simulink model "ship_template"  (R2021b)
settings: Solver=ode23t  StartTime=0.0  StopTime=60*2  MaxStep=0.1  RelTol=1e-3  AbsTol=1e-3
model workspace (MAT data in the model file):
  L = 1.2
  W = 1.2
undefined symbols (not defined in the file or in its folder): blue, blue0, blue1, blue2, centre, green, green0, green1, green2, left, Left, llx, lly, Mid, red, red0, red1, red2, right, Right, ulx, uly, X, Y, Z
libraries: sm_lib x278, nesl_utility x68, fl_lib x58, simulink x12, ee_lib x3, sdl_lib x3
(part 3 of 8)

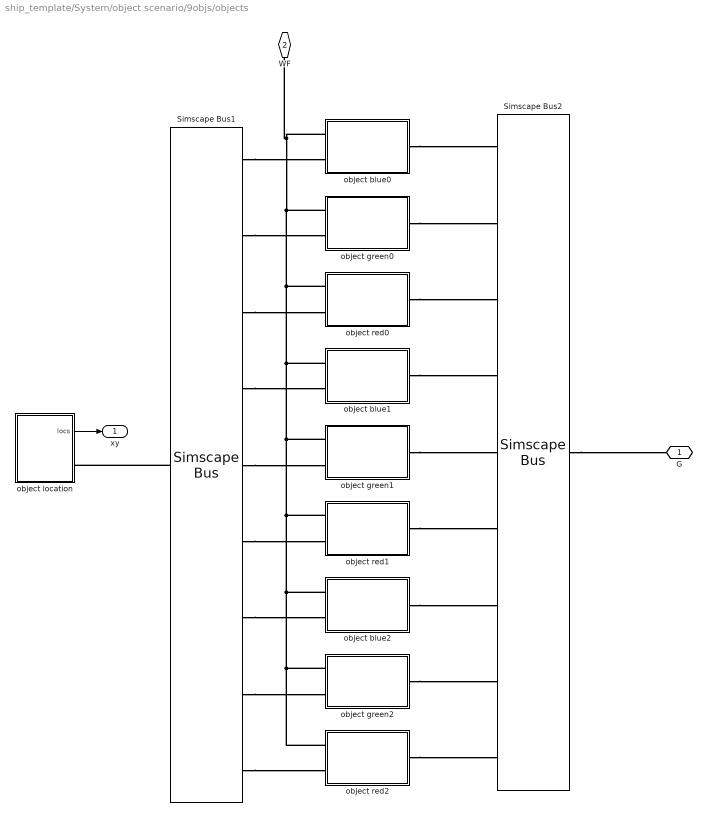
== system ship_template/System/object scenario/9objs/objects ==
  Simscape Bus1 : SimscapeBus  HierarchyStrings=blue0;green0;red0;blue1;green1;red1;blue2;green2;red2
  Simscape Bus2 : SimscapeBus  HierarchyStrings=blue0;green0;red0;blue1;green1;red1;blue2;green2;red2
  object blue0 : Subsystem  mask{x0=object_locs(1,1), y0=object_locs(1,2), color=[0.1 0.1 0.8]}
      mask prompts: x0 "Initial position x (m)"; y0 "Initial position y (m)"; color "Colour (RGB)"
  object blue1 : Subsystem  mask{x0=object_locs(4,1), y0=object_locs(4,2), color=[0.1 0.1 0.8]}
      mask prompts: x0 "Initial position x (m)"; y0 "Initial position y (m)"; color "Colour (RGB)"
  object blue2 : Subsystem  mask{x0=object_locs(7,1), y0=object_locs(7,2), color=[0.1 0.1 0.8]}
      mask prompts: x0 "Initial position x (m)"; y0 "Initial position y (m)"; color "Colour (RGB)"
  object green0 : Subsystem  mask{x0=object_locs(2,1), y0=object_locs(2,2), color=[0.1 0.8 0.1]}
      mask prompts: x0 "Initial position x (m)"; y0 "Initial position y (m)"; color "Colour (RGB)"
  object green1 : Subsystem  mask{x0=object_locs(5,1), y0=object_locs(5,2), color=[0.1 0.8 0.1]}
      mask prompts: x0 "Initial position x (m)"; y0 "Initial position y (m)"; color "Colour (RGB)"
  object green2 : Subsystem  mask{x0=object_locs(8,1), y0=object_locs(8,2), color=[0.1 0.8 0.1]}
      mask prompts: x0 "Initial position x (m)"; y0 "Initial position y (m)"; color "Colour (RGB)"
  object location : Subsystem  mask{Xhome=0, Yhome=0, homeRadius=0.1}
      mask prompts: Xhome "X home (m)"; Yhome "Y home (m)"; homeRadius "Home radius (m)"
  object red0 : Subsystem  mask{x0=object_locs(3,1), y0=object_locs(3,2), color=[0.8 0.1 0.1]}
      mask prompts: x0 "Initial position x (m)"; y0 "Initial position y (m)"; color "Colour (RGB)"
  object red1 : Subsystem  mask{x0=object_locs(6,1), y0=object_locs(6,2), color=[0.8 0.1 0.1]}
      mask prompts: x0 "Initial position x (m)"; y0 "Initial position y (m)"; color "Colour (RGB)"
  object red2 : Subsystem  mask{x0=object_locs(9,1), y0=object_locs(9,2), color=[0.8 0.1 0.1]}
      mask prompts: x0 "Initial position x (m)"; y0 "Initial position y (m)"; color "Colour (RGB)"
  G : PMIOPort  Side=Right
  WF : PMIOPort  Port=2  Side=Left
  xy : Outport
  wires:
  object location/1(locs) -> xy/1
  connections:
  object red0/RConn1 -- Simscape Bus2/LConn3
  object blue0/LConn1 -- object red2/LConn1 -- object green2/LConn1 -- object blue2/LConn1 -- object red1/LConn1 -- object green1/LConn1 -- object blue1/LConn1 -- object red0/LConn1 -- object green0/LConn1 -- WF/RConn1
  object blue0/RConn1 -- Simscape Bus2/LConn1
  object green0/RConn1 -- Simscape Bus2/LConn2
  Simscape Bus2/RConn1 -- G/RConn1
  Simscape Bus1/RConn1 -- object location/RConn1
  object blue1/RConn1 -- Simscape Bus2/LConn4
  object green1/RConn1 -- Simscape Bus2/LConn5
  object red1/RConn1 -- Simscape Bus2/LConn6
  object blue2/RConn1 -- Simscape Bus2/LConn7
  object green2/RConn1 -- Simscape Bus2/LConn8
  object red2/RConn1 -- Simscape Bus2/LConn9
  Simscape Bus1/LConn1 -- object blue0/LConn2
  Simscape Bus1/LConn2 -- object green0/LConn2
  Simscape Bus1/LConn3 -- object red0/LConn2
  Simscape Bus1/LConn4 -- object blue1/LConn2
  Simscape Bus1/LConn5 -- object green1/LConn2
  Simscape Bus1/LConn6 -- object red1/LConn2
  Simscape Bus1/LConn7 -- object blue2/LConn2
  Simscape Bus1/LConn8 -- object green2/LConn2
  Simscape Bus1/LConn9 -- object red2/LConn2

== system ship_template/System/propulsion and steering/one propeller and rudder (experimental)/Servo Rudder Mechanism ==
  angle : Inport
  Drag : Subsystem  mask{Cd=CdRud, L=LengthRudmm, D=DepthRudmm, rho=densityWorkingFluid}
      mask prompts: Cd "Drag coefficient"; L "Submerged Rudder Length (mm)"; D "Submerged Rudder Depth (mm)"; rho "Density"
  Pin : sm_lib/Body Elements/Cylindrical Solid  GraphicAmbientColor=[0.15 0.15 0.15 1.0]  BasedOnType=Density  CenterOfMass=[0 0 0]  CenterOfMassUnits=m  GraphicDiffuseColor=[1.0 1.0 1.0]  CylinderLength=5  CylinderLengthUnits=mm  CylinderRadius=3  CylinderRadiusUnits=mm  Density=1000  DensityUnits=kg/m^3  DoExposeReferenceFrame=on  GraphicEmissiveColor=[0.0 0.0 0.0 1.0]  ExportEntireGeometry=off  SerializedFrames=<Frames/>  MarkerShape=Sphere  MarkerSize=10  GraphicType=FromGeometry  InertiaType=CalculateFromGeometry  Mass=1  MassUnits=kg  MomentsOfInertia=[1 1 1]  MomentsOfInertiaUnits=kg*m^2  GraphicOpacity=1.0  ProductsOfInertia=[0 0 0]  ProductsOfInertiaUnits=kg*m^2  GraphicShininess=75  GraphicSpecularColor=[0.5 0.5 0.5 1.0]  GraphicVisPropType=SimpleVisualProperties
  Pin Rudder : sm_lib/Body Elements/Cylindrical Solid  GraphicAmbientColor=[0.15 0.15 0.15 1.0]  BasedOnType=Density  CenterOfMass=[0 0 0]  CenterOfMassUnits=m  GraphicDiffuseColor=[1.0 1.0 1.0]  CylinderLength=20  CylinderLengthUnits=mm  CylinderRadius=1  CylinderRadiusUnits=mm  Density=1000  DensityUnits=kg/m^3  DoExposeReferenceFrame=off  GraphicEmissiveColor=[0.0 0.0 0.0 1.0]  ExportEntireGeometry=off  SerializedFrames=<Frames><Frame><Id>Frame1</Id><Value><Name>F1</Name><Origin><Source>GeometricFeature</Source><FeatureName>top surface</FeatureName></Origin><PrimaryAxis><DefinedDirection>+Z</DefinedDirection><Source>ReferenceFrame</Source><SourceDirection>+Z</SourceDirection><FeatureName></FeatureName></PrimaryAxis><SecondaryAxis><DefinedDirection>+X</DefinedDirection><Source>ReferenceFrame</Source><SourceDirection>+X</SourceDirection><FeatureName></FeatureName></SecondaryAxis></Value></Frame></Frames>  MarkerShape=Sphere  MarkerSize=10  GraphicType=FromGeometry  InertiaType=CalculateFromGeometry  Mass=1  MassUnits=kg  MomentsOfInertia=[1 1 1]  MomentsOfInertiaUnits=kg*m^2  GraphicOpacity=1.0  ProductsOfInertia=[0 0 0]  ProductsOfInertiaUnits=kg*m^2  GraphicShininess=75  GraphicSpecularColor=[0.5 0.5 0.5 1.0]  GraphicVisPropType=SimpleVisualProperties
  Rigid Transform : sm_lib/Frames and Transforms/Rigid Transform  TranslationMethod=None  TranslationStandardOffset=0  TranslationLengthUnit=m  TranslationStandardAxis=+Z  TranslationCartesianOffset=[0 0 0]  TranslationROffset=0  TranslationROffsetUnits=m  TranslationZOffset=0  TranslationZOffsetUnits=m  TranslationThetaOffset=0  TranslationThetaOffsetUnits=deg  RotationMethod=None  RotationAngleUnits=deg  RotationStandardAxis=+Z  RotationAngle=0.0  RotationArbitraryAxis=[0 0 1]  FollAlignAxisA=+X  BaseAlignAxisA=+Y  FollAlignAxisB=+Y  BaseAlignAxisB=+Z  RotationSequenceAxes=FollowerAxes  RotationSequence=XYX  RotationSequenceAngles=[0 0 0]  RotationSequenceAnglesUnits=deg  RotationMatrix=[1 0 0; 0 1 0; 0 0 1]
  Rigid Transform1 : sm_lib/Frames and Transforms/Rigid Transform  TranslationMethod=None  TranslationStandardOffset=0  TranslationLengthUnit=m  TranslationStandardAxis=+Z  TranslationCartesianOffset=[0 0 0]  TranslationROffset=0  TranslationROffsetUnits=m  TranslationZOffset=0  TranslationZOffsetUnits=m  TranslationThetaOffset=0  TranslationThetaOffsetUnits=deg  RotationMethod=None  RotationAngleUnits=deg  RotationStandardAxis=+Z  RotationAngle=0.0  RotationArbitraryAxis=[0 0 1]  FollAlignAxisA=+X  BaseAlignAxisA=+Y  FollAlignAxisB=+Y  BaseAlignAxisB=+Z  RotationSequenceAxes=FollowerAxes  RotationSequence=XYX  RotationSequenceAngles=[0 0 0]  RotationSequenceAnglesUnits=deg  RotationMatrix=[1 0 0; 0 1 0; 0 0 1]
  Rigid Transform2 : sm_lib/Frames and Transforms/Rigid Transform  TranslationMethod=Cartesian  TranslationStandardOffset=50  TranslationLengthUnit=mm  TranslationStandardAxis=+X  TranslationCartesianOffset=[0 27 10]  TranslationROffset=0  TranslationROffsetUnits=m  TranslationZOffset=0  TranslationZOffsetUnits=m  TranslationThetaOffset=0  TranslationThetaOffsetUnits=deg  RotationMethod=None  RotationAngleUnits=deg  RotationStandardAxis=+Z  RotationAngle=0.0  RotationArbitraryAxis=[0 0 1]  FollAlignAxisA=+X  BaseAlignAxisA=+Y  FollAlignAxisB=+Y  BaseAlignAxisB=+Z  RotationSequenceAxes=FollowerAxes  RotationSequence=XYX  RotationSequenceAngles=[0 0 0]  RotationSequenceAnglesUnits=deg  RotationMatrix=[1 0 0; 0 1 0; 0 0 1]
  Servo : sm_lib/Body Elements/Brick Solid  GraphicAmbientColor=[0.15 0.15 0.15 1.0]  BasedOnType=Density  BrickDimensions=[20 10 20]  BrickDimensionUnits=mm  CenterOfMass=[0 0 0]  CenterOfMassUnits=m  GraphicDiffuseColor=[0.0 0.2 0.8]  Density=1000  DensityUnits=kg/m^3  DoExposeReferenceFrame=off  GraphicEmissiveColor=[0.0 0.0 0.0 1.0]  ExportEntireGeometry=off  SerializedFrames=<Frames><Frame><Id>Frame1</Id><Value><Name>+Z</Name><Origin><Source>GeometricFeature</Source><FeatureName>+z +x curve</FeatureName></Origin><PrimaryAxis><DefinedDirection>+Z</DefinedDirection><Source>ReferenceFrame</Source><SourceDirection>+Z</SourceDirection><FeatureName></FeatureName></PrimaryAxis><SecondaryAxis><DefinedDirection>+X</DefinedDirection><Source>ReferenceFrame</Source><SourceDirection>+X</SourceDirection><FeatureName></FeatureName></SecondaryAxis></Value></Frame></Frames>  MarkerShape=Sphere  MarkerSize=10  GraphicType=FromGeometry  InertiaType=CalculateFromGeometry  Mass=1  MassUnits=kg  MomentsOfInertia=[1 1 1]  MomentsOfInertiaUnits=kg*m^2  GraphicOpacity=1.0  ProductsOfInertia=[0 0 0]  ProductsOfInertiaUnits=kg*m^2  GraphicShininess=75  GraphicSpecularColor=[0.5 0.5 0.5 1.0]  GraphicVisPropType=SimpleVisualProperties
  Servo Axis : sm_lib/Joints/Revolute Joint  JointMode=Normal  SenseConstraintForce=off  SenseConstraintForceX=off  SenseConstraintForceY=off  SenseConstraintForceZ=off  SenseConstraintTorque=off  SenseConstraintTorqueX=off  SenseConstraintTorqueY=off  SenseConstraintTorqueZ=off  SenseTotalForce=off  SenseTotalForceX=off  SenseTotalForceY=off  SenseTotalForceZ=off  SenseTotalTorque=off  SenseTotalTorqueX=off  SenseTotalTorqueY=off  SenseTotalTorqueZ=off  CompositeWrenchDir=FollowerOnBase  CompositeWrenchFrame=BaseFrame  EquilibriumPosition=0  EquilibriumPositionUnits=deg  SpringStiffness=0  SpringStiffnessUnits=N*m/deg  DampingCoefficient=0  DampingCoefficientUnits=N*m/(deg/s)  TorqueActuationMode=ComputedTorque  MotionActuationMode=InputMotion  SensePosition=off  SenseVelocity=off  SenseAcceleration=off  SenseTorqueForce=off  SenseLowerLimitTorqueForce=off  SenseUpperLimitTorqueForce=off  LowerLimitSpecify=off  LowerLimitBound=-90  LowerLimitBoundUnits=deg  LowerLimitStiffness=1e4  LowerLimitStiffnessUnits=N*m/deg  LowerLimitDamping=10  LowerLimitDampingUnits=N*m/(deg/s)  LowerLimitTransitionRegionWidth=0.1  LowerLimitTransitionRegionWidthUnits=deg  UpperLimitSpecify=off  UpperLimitBound=90  UpperLimitBoundUnits=deg  UpperLimitStiffness=1e4  UpperLimitStiffnessUnits=N*m/deg  UpperLimitDamping=10  UpperLimitDampingUnits=N*m/(deg/s)  UpperLimitTransitionRegionWidth=0.1  UpperLimitTransitionRegionWidthUnits=deg  PositionTargetSpecify=off  PositionTargetPriority=High  PositionTargetValue=0  PositionTargetValueUnits=deg  VelocityTargetSpecify=off  VelocityTargetPriority=High  VelocityTargetValue=0  VelocityTargetValueUnits=deg/s
  Simulink-PS Converter : nesl_utility/Simulink-PS Converter  PhysicalDomain=network_engine_domain  SubClassName=ps_input  LeftPortType=input  RightPortType=output  PseudoPeriodic=off  Frequencies=[]  NoiseDistribution=none  NoiseParameters=[]  Unit=1  AffineConversion=off  FilteringAndDerivatives=filter  SimscapeFilterOrder=2  InputFilterTimeConstant=Tfilter  UdotUserProvided=0
      settings: SourceProductBaseCode=PW,SS
  hinge : sm_lib/Body Elements/Cylindrical Solid  GraphicAmbientColor=[0.15 0.15 0.15 1.0]  BasedOnType=Density  CenterOfMass=[0 0 0]  CenterOfMassUnits=m  GraphicDiffuseColor=[1.0 1.0 1.0]  CylinderLength=3  CylinderLengthUnits=mm  CylinderRadius=2  CylinderRadiusUnits=mm  Density=1000  DensityUnits=kg/m^3  DoExposeReferenceFrame=on  GraphicEmissiveColor=[0.0 0.0 0.0 1.0]  ExportEntireGeometry=off  SerializedFrames=<Frames/>  MarkerShape=Sphere  MarkerSize=10  GraphicType=FromGeometry  InertiaType=CalculateFromGeometry  Mass=1  MassUnits=kg  MomentsOfInertia=[1 1 1]  MomentsOfInertiaUnits=kg*m^2  GraphicOpacity=1.0  ProductsOfInertia=[0 0 0]  ProductsOfInertiaUnits=kg*m^2  GraphicShininess=75  GraphicSpecularColor=[0.5 0.5 0.5 1.0]  GraphicVisPropType=SimpleVisualProperties
  lever arm : sm_lib/Body Elements/Brick Solid  GraphicAmbientColor=[0.15 0.15 0.15 1.0]  BasedOnType=Density  BrickDimensions=[15 2 2]  BrickDimensionUnits=mm  CenterOfMass=[0 0 0]  CenterOfMassUnits=m  GraphicDiffuseColor=[0.5 0.5 0.5]  Density=1000  DensityUnits=kg/m^3  DoExposeReferenceFrame=off  GraphicEmissiveColor=[0.0 0.0 0.0 1.0]  ExportEntireGeometry=off  SerializedFrames=<Frames><Frame><Id>Frame1</Id><Value><Name>+X</Name><Origin><Source>GeometricFeature</Source><FeatureName>+x surface</FeatureName></Origin><PrimaryAxis><DefinedDirection>+Z</DefinedDirection><Source>ReferenceFrame</Source><SourceDirection>+Z</SourceDirection><FeatureName></FeatureName></PrimaryAxis><SecondaryAxis><DefinedDirection>+X</DefinedDirection><Source>ReferenceFrame</Source><SourceDirection>+X</SourceDirection><FeatureName></FeatureName></SecondaryAxis></Value></Frame><Frame><Id>Frame2</Id><Value><Name>-X</Name><Origin><Source>GeometricFeature</Source><FeatureName>-x surface</FeatureName></Origin><PrimaryAxis><DefinedDirection>+Z</DefinedDirection><Source>ReferenceFrame</Source><SourceDirection>+Z</SourceDirection><FeatureName></FeatureName></PrimaryAxis><SecondaryAxis><DefinedDirection>+X</DefinedDirection><Source>ReferenceFrame</Source><SourceDirection>+X</SourceDirection><FeatureName></FeatureName></SecondaryAxis></Value></Frame></Frames>  MarkerShape=Sphere  MarkerSize=10  GraphicType=FromGeometry  InertiaType=CalculateFromGeometry  Mass=1  MassUnits=kg  MomentsOfInertia=[1 1 1]  MomentsOfInertiaUnits=kg*m^2  GraphicOpacity=1.0  ProductsOfInertia=[0 0 0]  ProductsOfInertiaUnits=kg*m^2  GraphicShininess=75  GraphicSpecularColor=[0.5 0.5 0.5 1.0]  GraphicVisPropType=SimpleVisualProperties
  B : PMIOPort  Side=Right
  wires:
  angle/1 -> Simulink-PS Converter/1
  connections:
  Rigid Transform2/RConn1 -- Pin/RConn1 -- Servo/LConn1 -- Rigid Transform/LConn1
  Drag/LConn1 -- lever arm/LConn1 -- Pin Rudder/LConn1 -- hinge/RConn1
  Servo Axis/RConn1 -- Rigid Transform1/LConn1
  Servo Axis/LConn2 -- Simulink-PS Converter/RConn1
  lever arm/RConn1 -- Rigid Transform1/RConn1
  Servo Axis/LConn1 -- Rigid Transform/RConn1
  B/RConn1 -- Rigid Transform2/LConn1

== system ship_template/System/propulsion and steering/one propeller and rudder (experimental)/Ship Locations ==
  Motor : Subsystem
  Simscape Bus : SimscapeBus  HierarchyStrings=Mid;Left;Right
  Prop Axis : PMIOPort  Side=Left
  Props : PMIOPort  Port=2  Side=Right
  Base : PMIOPort  Port=3  Side=Left
  connections:
  Simscape Bus/RConn1 -- Props/RConn1
  Simscape Bus/LConn1 -- Base/RConn1 -- Motor/LConn1
  Motor/RConn1 -- Prop Axis/RConn1

== system ship_template/System/propulsion and steering/one propeller and rudder (experimental)/motor mixer ==
  v : Inport
  w : Inport  Port=2
  Bias : Bias  Bias=0.0
  Gain : Gain  Gain=0.1
  Gain1 : Gain  Gain=pi/4
  Saturation : Saturate  UpperLimit=pi/4  LowerLimit=-pi/4
  PWM : Outport
  angle : Outport  Port=2
  wires:
  Bias/1 -> Saturation/1
  v/1 -> Gain/1
  Gain/1 -> PWM/1
  w/1 -> Gain1/1
  Gain1/1 -> Bias/1
  Saturation/1 -> angle/1

== system ship_template/System/propulsion and steering/one propeller and rudder (experimental)/propeller thrust model ==
  PWM : Inport
  lookup model : Subsystem  VariantControl=lookup
  physical model : Subsystem  VariantControl=physmod
  simple thrust : Subsystem  VariantControl=gain
  simulink model : Subsystem  VariantControl=ode
  thrust : PMIOPort  Side=Right

== system ship_template/System/propulsion and steering/two propeller/Propellers ==
  DC_Motor_1 : Subsystem
  DC_Motor_2 : Subsystem
  Mixer_Propeller_1 : Subsystem
  Mixer_Propeller_2 : Subsystem
  Rev1 : sm_lib/Joints/Revolute Joint  JointMode=Normal  SenseConstraintForce=off  SenseConstraintForceX=off  SenseConstraintForceY=off  SenseConstraintForceZ=off  SenseConstraintTorque=off  SenseConstraintTorqueX=off  SenseConstraintTorqueY=off  SenseConstraintTorqueZ=off  SenseTotalForce=off  SenseTotalForceX=off  SenseTotalForceY=off  SenseTotalForceZ=off  SenseTotalTorque=off  SenseTotalTorqueX=off  SenseTotalTorqueY=off  SenseTotalTorqueZ=off  CompositeWrenchDir=FollowerOnBase  CompositeWrenchFrame=BaseFrame  EquilibriumPosition=0  EquilibriumPositionUnits=deg  SpringStiffness=0  SpringStiffnessUnits=N*m/deg  DampingCoefficient=0  DampingCoefficientUnits=kg*m^2/(rad*s)  TorqueActuationMode=ComputedTorque  MotionActuationMode=InputMotion  SensePosition=off  SenseVelocity=off  SenseAcceleration=off  SenseTorqueForce=off  SenseLowerLimitTorqueForce=off  SenseUpperLimitTorqueForce=off  LowerLimitSpecify=off  LowerLimitBound=-90  LowerLimitBoundUnits=deg  LowerLimitStiffness=1e4  LowerLimitStiffnessUnits=N*m/deg  LowerLimitDamping=10  LowerLimitDampingUnits=N*m/(deg/s)  LowerLimitTransitionRegionWidth=0.1  LowerLimitTransitionRegionWidthUnits=deg  UpperLimitSpecify=off  UpperLimitBound=90  UpperLimitBoundUnits=deg  UpperLimitStiffness=1e4  UpperLimitStiffnessUnits=N*m/deg  UpperLimitDamping=10  UpperLimitDampingUnits=N*m/(deg/s)  UpperLimitTransitionRegionWidth=0.1  UpperLimitTransitionRegionWidthUnits=deg  PositionTargetSpecify=off  PositionTargetPriority=High  PositionTargetValue=0  PositionTargetValueUnits=deg  VelocityTargetSpecify=off  VelocityTargetPriority=High  VelocityTargetValue=0  VelocityTargetValueUnits=deg/s
  Rev2 : sm_lib/Joints/Revolute Joint  JointMode=Normal  SenseConstraintForce=off  SenseConstraintForceX=off  SenseConstraintForceY=off  SenseConstraintForceZ=off  SenseConstraintTorque=off  SenseConstraintTorqueX=off  SenseConstraintTorqueY=off  SenseConstraintTorqueZ=off  SenseTotalForce=off  SenseTotalForceX=off  SenseTotalForceY=off  SenseTotalForceZ=off  SenseTotalTorque=off  SenseTotalTorqueX=off  SenseTotalTorqueY=off  SenseTotalTorqueZ=off  CompositeWrenchDir=FollowerOnBase  CompositeWrenchFrame=BaseFrame  EquilibriumPosition=0  EquilibriumPositionUnits=deg  SpringStiffness=0  SpringStiffnessUnits=N*m/deg  DampingCoefficient=0  DampingCoefficientUnits=kg*m^2/(rad*s)  TorqueActuationMode=ComputedTorque  MotionActuationMode=InputMotion  SensePosition=off  SenseVelocity=off  SenseAcceleration=off  SenseTorqueForce=off  SenseLowerLimitTorqueForce=off  SenseUpperLimitTorqueForce=off  LowerLimitSpecify=off  LowerLimitBound=-90  LowerLimitBoundUnits=deg  LowerLimitStiffness=1e4  LowerLimitStiffnessUnits=N*m/deg  LowerLimitDamping=10  LowerLimitDampingUnits=N*m/(deg/s)  LowerLimitTransitionRegionWidth=0.1  LowerLimitTransitionRegionWidthUnits=deg  UpperLimitSpecify=off  UpperLimitBound=90  UpperLimitBoundUnits=deg  UpperLimitStiffness=1e4  UpperLimitStiffnessUnits=N*m/deg  UpperLimitDamping=10  UpperLimitDampingUnits=N*m/(deg/s)  UpperLimitTransitionRegionWidth=0.1  UpperLimitTransitionRegionWidthUnits=deg  PositionTargetSpecify=off  PositionTargetPriority=High  PositionTargetValue=0  PositionTargetValueUnits=deg  VelocityTargetSpecify=off  VelocityTargetPriority=High  VelocityTargetValue=0  VelocityTargetValueUnits=deg/s
  Rigid3 : sm_lib/Joints/Weld Joint  JointMode=Normal  SenseConstraintForce=off  SenseConstraintForceX=off  SenseConstraintForceY=off  SenseConstraintForceZ=off  SenseConstraintTorque=off  SenseConstraintTorqueX=off  SenseConstraintTorqueY=off  SenseConstraintTorqueZ=off  SenseTotalForce=on  SenseTotalForceX=off  SenseTotalForceY=off  SenseTotalForceZ=off  SenseTotalTorque=off  SenseTotalTorqueX=off  SenseTotalTorqueY=off  SenseTotalTorqueZ=off  CompositeWrenchDir=FollowerOnBase  CompositeWrenchFrame=BaseFrame
  Rigid4 : sm_lib/Joints/Weld Joint  JointMode=Normal  SenseConstraintForce=off  SenseConstraintForceX=off  SenseConstraintForceY=off  SenseConstraintForceZ=off  SenseConstraintTorque=off  SenseConstraintTorqueX=off  SenseConstraintTorqueY=off  SenseConstraintTorqueZ=off  SenseTotalForce=on  SenseTotalForceX=off  SenseTotalForceY=off  SenseTotalForceZ=off  SenseTotalTorque=off  SenseTotalTorqueX=off  SenseTotalTorqueY=off  SenseTotalTorqueZ=off  CompositeWrenchDir=FollowerOnBase  CompositeWrenchFrame=BaseFrame
  Simscape Bus : SimscapeBus  HierarchyStrings=Mid;Left;Right
  animate1 : Subsystem
  animate2 : Subsystem
  PropLeft : PMIOPort  Side=Left
  PropRight : PMIOPort  Port=2  Side=Left
  Props : PMIOPort  Port=3  Side=Right
  connections:
  animate2/RConn1 -- Rev2/LConn2
  Rigid3/RConn1 -- DC_Motor_1/LConn1
  Rev1/RConn1 -- Mixer_Propeller_1/LConn1
  Rev2/LConn1 -- DC_Motor_2/RConn1 -- PropRight/RConn1
  Rigid4/RConn1 -- DC_Motor_2/LConn1
  Rev2/RConn1 -- Mixer_Propeller_2/LConn1
  Rev1/LConn1 -- DC_Motor_1/RConn1 -- PropLeft/RConn1
  Rigid4/RConn2 -- animate2/LConn1
  animate1/LConn1 -- Rigid3/RConn2
  animate1/RConn1 -- Rev1/LConn2
  Simscape Bus/LConn2 -- Rigid3/LConn1
  Simscape Bus/RConn1 -- Props/RConn1
  Simscape Bus/LConn3 -- Rigid4/LConn1

== system ship_template/System/propulsion and steering/two propeller/motor mixer ==
  v : Inport
  w : Inport  Port=2
  Sum : Sum
  Sum1 : Sum  Inputs=-+
  PWM_left : Outport
  PWM_right : Outport  Port=2
  wires:
  Sum/1 -> PWM_left/1
  Sum1/1 -> PWM_right/1
  w/1 -> Sum/2, Sum1/1
  v/1 -> Sum1/2, Sum/1

== system ship_template/System/propulsion and steering/two propeller/propeller thrust model ==
  PWM_left : Inport
  PWM_right : Inport  Port=2
  lookup model : Subsystem  VariantControl=lookup
  physical model : Subsystem  VariantControl=physmod
  simple thrust : Subsystem  VariantControl=gain
  simulink model : Subsystem  VariantControl=ode
  thrust_left : PMIOPort  Side=Right
  thrust_right : PMIOPort  Port=2  Side=Right

== system ship_template/System/ship to world joint/nonlinear_drag/Drag model ==
  External Force and Torque : sm_lib/Forces and Torques/External Force and Torque  ForceResolutionFrame=World  EnableForceX=on  EnableForceY=on  EnableForceZ=off  EnableForce=off  TorqueResolutionFrame=AttachedFrame  EnableTorqueX=off  EnableTorqueY=off  EnableTorqueZ=on  EnableTorque=off
  PS Gain : fl_lib/Physical Signals/Functions/PS Gain  gain=-1
  PS Gain1 : fl_lib/Physical Signals/Functions/PS Gain  gain=-1
  PS Gain2 : fl_lib/Physical Signals/Functions/PS Gain  gain=-1
  rotational_drag_model_theta : Subsystem  mask{Cd=0.05, rho=1000, A=60*120e-6, R=6e-3}
      mask prompts: Cd "Drag Coefficient"; rho "Density"; A "Project Area"; R "Moment Arm"
  translational_drag_model_x : Subsystem  mask{Cd=0.4, rho=1000, A=60*20e-6}
      mask prompts: Cd "Drag Coefficient"; rho "Density"; A "Project Area"
  translational_drag_model_y : Subsystem  mask{Cd=0.4, rho=1000, A=60*120e-6}
      mask prompts: Cd "Drag Coefficient"; rho "Density"; A "Project Area"
  F : PMIOPort  Side=Left
  vx : PMIOPort  Port=2  Side=Left
  vy : PMIOPort  Port=3  Side=Left
  wz : PMIOPort  Port=4  Side=Left
  connections:
  External Force and Torque/RConn1 -- F/RConn1
  vy/RConn1 -- translational_drag_model_y/LConn1
  rotational_drag_model_theta/RConn1 -- PS Gain2/LConn1
  PS Gain/LConn1 -- translational_drag_model_x/RConn1
  translational_drag_model_x/LConn1 -- vx/RConn1
  translational_drag_model_y/RConn1 -- PS Gain1/LConn1
  wz/RConn1 -- rotational_drag_model_theta/LConn1
  PS Gain/RConn1 -- External Force and Torque/LConn1
  External Force and Torque/LConn2 -- PS Gain1/RConn1
  PS Gain2/RConn1 -- External Force and Torque/LConn3

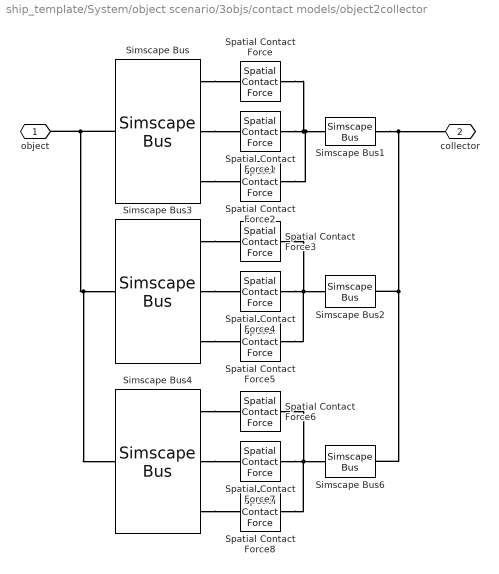
== system ship_template/System/object scenario/3objs/contact models/object2collector ==
  Simscape Bus : SimscapeBus  HierarchyStrings=blue;green;red
  Simscape Bus1 : SimscapeBus  HierarchyStrings=left
  Simscape Bus2 : SimscapeBus  HierarchyStrings=centre
  Simscape Bus3 : SimscapeBus  HierarchyStrings=blue;green;red
  Simscape Bus4 : SimscapeBus  HierarchyStrings=blue;green;red
  Simscape Bus6 : SimscapeBus  HierarchyStrings=right
  Spatial Contact Force{,1..8} (9 alike) : sm_lib/Forces and Torques/Spatial Contact Force  CoefficientOfDynamicFriction=0.3  CoefficientOfStaticFriction=0.5  SenseContactBaseRotation=off  SenseContactBaseTranslation=off  NormalDamping=b  NormalDampingUnits=N/(m/s)  SenseContactFollowerRotation=off  SenseContactFollowerTranslation=off  SenseContactSignal=off  NormalStiffness=k  NormalStiffnessUnits=N/m  FrictionalCriticalVelocity=1e-3  FrictionalCriticalVelocityUnits=m/s  ZeroCrossDetectContactStartAndEnd=on  FrictionType=SmoothStickSlip  SenseFrictionalForceMagnitude=off  SenseNormalForceMagnitude=off  NormalForceType=SmoothSpringDamper  SenseNormalVelocity=off  SenseSeparationDistance=off  SenseTangentialVelocity=off  SenseTangentialVelocityMagnitude=off  NormalTransitionRegionWidth=x  NormalTransitionRegionWidthUnits=m
  object : PMIOPort  Side=Left
  collector : PMIOPort  Port=2  Side=Right
  connections:
  Simscape Bus3/LConn1 -- Spatial Contact Force3/LConn1
  Simscape Bus/LConn3 -- Spatial Contact Force2/LConn1
  Simscape Bus/LConn1 -- Spatial Contact Force/LConn1
  Spatial Contact Force/RConn1 -- Spatial Contact Force2/RConn1 -- Simscape Bus1/LConn1 -- Spatial Contact Force1/RConn1
  Simscape Bus/LConn2 -- Spatial Contact Force1/LConn1
  Simscape Bus/RConn1 -- object/RConn1 -- Simscape Bus4/RConn1 -- Simscape Bus3/RConn1
  Spatial Contact Force6/RConn1 -- Simscape Bus6/LConn1 -- Spatial Contact Force8/RConn1 -- Spatial Contact Force7/RConn1
  Simscape Bus4/LConn3 -- Spatial Contact Force8/LConn1
  Simscape Bus4/LConn2 -- Spatial Contact Force7/LConn1
  Simscape Bus1/RConn1 -- collector/RConn1 -- Simscape Bus6/RConn1 -- Simscape Bus2/RConn1
  Spatial Contact Force5/RConn1 -- Spatial Contact Force3/RConn1 -- Simscape Bus2/LConn1 -- Spatial Contact Force4/RConn1
  Simscape Bus4/LConn1 -- Spatial Contact Force6/LConn1
  Simscape Bus3/LConn3 -- Spatial Contact Force5/LConn1
  Simscape Bus3/LConn2 -- Spatial Contact Force4/LConn1

== system ship_template/System/object scenario/3objs/contact models/object2object ==
  Simscape Bus10 : SimscapeBus  HierarchyStrings=green
  Simscape Bus7 : SimscapeBus  HierarchyStrings=green;red
  Simscape Bus8 : SimscapeBus  HierarchyStrings=blue
  Simscape Bus9 : SimscapeBus  HierarchyStrings=red
  Spatial Contact Force13 : sm_lib/Forces and Torques/Spatial Contact Force  CoefficientOfDynamicFriction=0.3  CoefficientOfStaticFriction=0.5  SenseContactBaseRotation=off  SenseContactBaseTranslation=off  NormalDamping=b  NormalDampingUnits=N/(m/s)  SenseContactFollowerRotation=off  SenseContactFollowerTranslation=off  SenseContactSignal=off  NormalStiffness=k  NormalStiffnessUnits=N/m  FrictionalCriticalVelocity=1e-3  FrictionalCriticalVelocityUnits=m/s  ZeroCrossDetectContactStartAndEnd=off  FrictionType=SmoothStickSlip  SenseFrictionalForceMagnitude=off  SenseNormalForceMagnitude=off  NormalForceType=SmoothSpringDamper  SenseNormalVelocity=off  SenseSeparationDistance=off  SenseTangentialVelocity=off  SenseTangentialVelocityMagnitude=off  NormalTransitionRegionWidth=x  NormalTransitionRegionWidthUnits=m
  Spatial Contact Force14 : sm_lib/Forces and Torques/Spatial Contact Force  CoefficientOfDynamicFriction=0.3  CoefficientOfStaticFriction=0.5  SenseContactBaseRotation=off  SenseContactBaseTranslation=off  NormalDamping=b  NormalDampingUnits=N/(m/s)  SenseContactFollowerRotation=off  SenseContactFollowerTranslation=off  SenseContactSignal=off  NormalStiffness=k  NormalStiffnessUnits=N/m  FrictionalCriticalVelocity=1e-3  FrictionalCriticalVelocityUnits=m/s  ZeroCrossDetectContactStartAndEnd=off  FrictionType=SmoothStickSlip  SenseFrictionalForceMagnitude=off  SenseNormalForceMagnitude=off  NormalForceType=SmoothSpringDamper  SenseNormalVelocity=off  SenseSeparationDistance=off  SenseTangentialVelocity=off  SenseTangentialVelocityMagnitude=off  NormalTransitionRegionWidth=x  NormalTransitionRegionWidthUnits=m
  Spatial Contact Force15 : sm_lib/Forces and Torques/Spatial Contact Force  CoefficientOfDynamicFriction=0.3  CoefficientOfStaticFriction=0.5  SenseContactBaseRotation=off  SenseContactBaseTranslation=off  NormalDamping=b  NormalDampingUnits=N/(m/s)  SenseContactFollowerRotation=off  SenseContactFollowerTranslation=off  SenseContactSignal=off  NormalStiffness=k  NormalStiffnessUnits=N/m  FrictionalCriticalVelocity=1e-3  FrictionalCriticalVelocityUnits=m/s  ZeroCrossDetectContactStartAndEnd=off  FrictionType=SmoothStickSlip  SenseFrictionalForceMagnitude=off  SenseNormalForceMagnitude=off  NormalForceType=SmoothSpringDamper  SenseNormalVelocity=off  SenseSeparationDistance=off  SenseTangentialVelocity=off  SenseTangentialVelocityMagnitude=off  NormalTransitionRegionWidth=x  NormalTransitionRegionWidthUnits=m
  object : PMIOPort  Side=Left
  connections:
  Spatial Contact Force15/RConn1 -- Simscape Bus10/LConn1
  Simscape Bus7/RConn1 -- object/RConn1 -- Simscape Bus9/RConn1 -- Simscape Bus8/RConn1 -- Simscape Bus10/RConn1
  Spatial Contact Force13/RConn1 -- Spatial Contact Force14/RConn1 -- Simscape Bus8/LConn1
  Simscape Bus7/LConn1 -- Spatial Contact Force13/LConn1
  Spatial Contact Force15/LConn1 -- Simscape Bus9/LConn1
  Spatial Contact Force14/LConn1 -- Simscape Bus7/LConn2

== system ship_template/System/object scenario/3objs/contact models/object2ship ==
  Simscape Bus5 : SimscapeBus  HierarchyStrings=blue;green;red
  Spatial Contact Force10 : sm_lib/Forces and Torques/Spatial Contact Force  CoefficientOfDynamicFriction=0.3  CoefficientOfStaticFriction=0.5  SenseContactBaseRotation=off  SenseContactBaseTranslation=off  NormalDamping=b  NormalDampingUnits=N/(m/s)  SenseContactFollowerRotation=off  SenseContactFollowerTranslation=off  SenseContactSignal=off  NormalStiffness=k  NormalStiffnessUnits=N/m  FrictionalCriticalVelocity=1e-3  FrictionalCriticalVelocityUnits=m/s  ZeroCrossDetectContactStartAndEnd=off  FrictionType=SmoothStickSlip  SenseFrictionalForceMagnitude=off  SenseNormalForceMagnitude=off  NormalForceType=SmoothSpringDamper  SenseNormalVelocity=off  SenseSeparationDistance=off  SenseTangentialVelocity=off  SenseTangentialVelocityMagnitude=off  NormalTransitionRegionWidth=x  NormalTransitionRegionWidthUnits=m
  Spatial Contact Force11 : sm_lib/Forces and Torques/Spatial Contact Force  CoefficientOfDynamicFriction=0.3  CoefficientOfStaticFriction=0.5  SenseContactBaseRotation=off  SenseContactBaseTranslation=off  NormalDamping=b  NormalDampingUnits=N/(m/s)  SenseContactFollowerRotation=off  SenseContactFollowerTranslation=off  SenseContactSignal=off  NormalStiffness=k  NormalStiffnessUnits=N/m  FrictionalCriticalVelocity=1e-3  FrictionalCriticalVelocityUnits=m/s  ZeroCrossDetectContactStartAndEnd=off  FrictionType=SmoothStickSlip  SenseFrictionalForceMagnitude=off  SenseNormalForceMagnitude=off  NormalForceType=SmoothSpringDamper  SenseNormalVelocity=off  SenseSeparationDistance=off  SenseTangentialVelocity=off  SenseTangentialVelocityMagnitude=off  NormalTransitionRegionWidth=x  NormalTransitionRegionWidthUnits=m
  Spatial Contact Force9 : sm_lib/Forces and Torques/Spatial Contact Force  CoefficientOfDynamicFriction=0.3  CoefficientOfStaticFriction=0.5  SenseContactBaseRotation=off  SenseContactBaseTranslation=off  NormalDamping=b  NormalDampingUnits=N/(m/s)  SenseContactFollowerRotation=off  SenseContactFollowerTranslation=off  SenseContactSignal=off  NormalStiffness=k  NormalStiffnessUnits=N/m  FrictionalCriticalVelocity=1e-3  FrictionalCriticalVelocityUnits=m/s  ZeroCrossDetectContactStartAndEnd=off  FrictionType=SmoothStickSlip  SenseFrictionalForceMagnitude=off  SenseNormalForceMagnitude=off  NormalForceType=SmoothSpringDamper  SenseNormalVelocity=off  SenseSeparationDistance=off  SenseTangentialVelocity=off  SenseTangentialVelocityMagnitude=off  NormalTransitionRegionWidth=x  NormalTransitionRegionWidthUnits=m
  object : PMIOPort  Side=Left
  ship : PMIOPort  Port=2  Side=Right
  connections:
  Simscape Bus5/LConn3 -- Spatial Contact Force11/LConn1
  Spatial Contact Force9/LConn1 -- Simscape Bus5/LConn1
  Spatial Contact Force11/RConn1 -- ship/RConn1 -- Spatial Contact Force9/RConn1 -- Spatial Contact Force10/RConn1
  Simscape Bus5/LConn2 -- Spatial Contact Force10/LConn1
  object/RConn1 -- Simscape Bus5/RConn1

== system ship_template/System/object scenario/3objs/contact models/tank2collector ==
  Simscape Bus1 : SimscapeBus  HierarchyStrings=left
  Simscape Bus2 : SimscapeBus  HierarchyStrings=centre
  Simscape Bus6 : SimscapeBus  HierarchyStrings=right
  Subsystem : Subsystem
  Subsystem1 : Subsystem
  Subsystem2 : Subsystem
  tank wall : PMIOPort  Side=Left
  collector : PMIOPort  Port=2  Side=Right
  connections:
  tank wall/RConn1 -- Subsystem1/LConn1 -- Subsystem2/LConn1 -- Subsystem/LConn1
  Simscape Bus2/RConn1 -- Simscape Bus1/RConn1 -- collector/RConn1 -- Simscape Bus6/RConn1
  Subsystem/RConn1 -- Simscape Bus1/LConn1
  Subsystem2/RConn1 -- Simscape Bus6/LConn1
  Subsystem1/RConn1 -- Simscape Bus2/LConn1

== system ship_template/System/object scenario/3objs/objects/object blue ==
  External Force and Torque : sm_lib/Forces and Torques/External Force and Torque  ForceResolutionFrame=AttachedFrame  EnableForceX=on  EnableForceY=off  EnableForceZ=off  EnableForce=off  TorqueResolutionFrame=AttachedFrame  EnableTorqueX=off  EnableTorqueY=off  EnableTorqueZ=off  EnableTorque=off
  PS Constant : fl_lib/Physical Signals/Sources/PS Constant  constant=f
  Rectangular Joint : sm_lib/Joints/Rectangular Joint  JointMode=Normal  SenseConstraintForce=off  SenseConstraintForceX=off  SenseConstraintForceY=off  SenseConstraintForceZ=off  SenseConstraintTorque=off  SenseConstraintTorqueX=off  SenseConstraintTorqueY=off  SenseConstraintTorqueZ=off  SenseTotalForce=off  SenseTotalForceX=off  SenseTotalForceY=off  SenseTotalForceZ=off  SenseTotalTorque=off  SenseTotalTorqueX=off  SenseTotalTorqueY=off  SenseTotalTorqueZ=off  CompositeWrenchDir=FollowerOnBase  CompositeWrenchFrame=BaseFrame  PxEquilibriumPosition=0  PxEquilibriumPositionUnits=m  PxSpringStiffness=0  PxSpringStiffnessUnits=N/m  PxDampingCoefficient=b  PxDampingCoefficientUnits=N/(m/s)  PxTorqueActuationMode=NoTorque  PxMotionActuationMode=ComputedMotion  PxSensePosition=off  PxSenseVelocity=off  PxSenseAcceleration=off  PxSenseTorqueForce=off  PxSenseLowerLimitTorqueForce=off  PxSenseUpperLimitTorqueForce=off  PxLowerLimitSpecify=on  PxLowerLimitBound=-L/2  PxLowerLimitBoundUnits=m  PxLowerLimitStiffness=1e5  PxLowerLimitStiffnessUnits=N/m  PxLowerLimitDamping=sqrt(2e5)  PxLowerLimitDampingUnits=N/(m/s)  PxLowerLimitTransitionRegionWidth=1e-3  PxLowerLimitTransitionRegionWidthUnits=m  PxUpperLimitSpecify=on  PxUpperLimitBound=L/2  PxUpperLimitBoundUnits=m  PxUpperLimitStiffness=1e4  PxUpperLimitStiffnessUnits=N/m  PxUpperLimitDamping=sqrt(2e5)  PxUpperLimitDampingUnits=N/(m/s)  PxUpperLimitTransitionRegionWidth=1e-3  PxUpperLimitTransitionRegionWidthUnits=m  PxPositionTargetSpecify=on  PxPositionTargetPriority=High  PxPositionTargetValue=x0  PxPositionTargetValueUnits=m  PxVelocityTargetSpecify=off  PxVelocityTargetPriority=High  PxVelocityTargetValue=0  PxVelocityTargetValueUnits=m/s  PyEquilibriumPosition=0  PyEquilibriumPositionUnits=m  PySpringStiffness=0  PySpringStiffnessUnits=N/m  PyDampingCoefficient=b  PyDampingCoefficientUnits=N/(m/s)  PyTorqueActuationMode=NoTorque  PyMotionActuationMode=ComputedMotion  PySensePosition=off  PySenseVelocity=off  PySenseAcceleration=off  PySenseTorqueForce=off  PySenseLowerLimitTorqueForce=off  PySenseUpperLimitTorqueForce=off  PyLowerLimitSpecify=on  PyLowerLimitBound=-W/2  PyLowerLimitBoundUnits=m  PyLowerLimitStiffness=1e5  PyLowerLimitStiffnessUnits=N/m  PyLowerLimitDamping=sqrt(2e5)  PyLowerLimitDampingUnits=N/(m/s)  PyLowerLimitTransitionRegionWidth=1e-3  PyLowerLimitTransitionRegionWidthUnits=m  PyUpperLimitSpecify=on  PyUpperLimitBound=W/2  PyUpperLimitBoundUnits=m  PyUpperLimitStiffness=1e5  PyUpperLimitStiffnessUnits=N/m  PyUpperLimitDamping=sqrt(2e5)  PyUpperLimitDampingUnits=N/(m/s)  PyUpperLimitTransitionRegionWidth=1e-3  PyUpperLimitTransitionRegionWidthUnits=m  PyPositionTargetSpecify=on  PyPositionTargetPriority=High  PyPositionTargetValue=y0  PyPositionTargetValueUnits=m  PyVelocityTargetSpecify=off  PyVelocityTargetPriority=High  PyVelocityTargetValue=0  PyVelocityTargetValueUnits=m/s
  Spherical Solid : sm_lib/Body Elements/Spherical Solid  GraphicAmbientColor=[0.15 0.15 0.15 1.0]  BasedOnType=Density  CenterOfMass=[0 0 0]  CenterOfMassUnits=m  GraphicDiffuseColor=color  Density=1000  DensityUnits=kg/m^3  DoExposeReferenceFrame=on  GraphicEmissiveColor=[0.0 0.0 0.0 1.0]  ExportEntireGeometry=on  SerializedExposedGeometries=<ExposedGeometries><ExposedGeometry><RawGeometryId>entire</RawGeometryId><ExposedGeometryId>G</ExposedGeometryId></ExposedGeometry></ExposedGeometries>  SerializedFrames=<Frames/>  MarkerShape=Sphere  MarkerSize=10  GraphicType=FromGeometry  InertiaType=CalculateFromGeometry  Mass=1  MassUnits=kg  MomentsOfInertia=[1 1 1]  MomentsOfInertiaUnits=kg*m^2  GraphicOpacity=1.0  ProductsOfInertia=[0 0 0]  ProductsOfInertiaUnits=kg*m^2  GraphicShininess=75  GraphicSpecularColor=[0.5 0.5 0.5 1.0]  SphereRadius=R  SphereRadiusUnits=mm  GraphicVisPropType=SimpleVisualProperties
  WF : PMIOPort  Side=Left
  G : PMIOPort  Port=2  Side=Right
  R : PMIOPort  Port=3  Side=Left
  connections:
  PS Constant/RConn1 -- External Force and Torque/LConn1
  External Force and Torque/RConn1 -- Rectangular Joint/RConn1 -- R/RConn1 -- Spherical Solid/RConn1
  Spherical Solid/LConn1 -- G/RConn1
  Rectangular Joint/LConn1 -- WF/RConn1

== system ship_template/System/object scenario/3objs/objects/object green ==
  External Force and Torque : sm_lib/Forces and Torques/External Force and Torque  ForceResolutionFrame=AttachedFrame  EnableForceX=on  EnableForceY=off  EnableForceZ=off  EnableForce=off  TorqueResolutionFrame=AttachedFrame  EnableTorqueX=off  EnableTorqueY=off  EnableTorqueZ=off  EnableTorque=off
  PS Constant : fl_lib/Physical Signals/Sources/PS Constant  constant=f
  Rectangular Joint : sm_lib/Joints/Rectangular Joint  JointMode=Normal  SenseConstraintForce=off  SenseConstraintForceX=off  SenseConstraintForceY=off  SenseConstraintForceZ=off  SenseConstraintTorque=off  SenseConstraintTorqueX=off  SenseConstraintTorqueY=off  SenseConstraintTorqueZ=off  SenseTotalForce=off  SenseTotalForceX=off  SenseTotalForceY=off  SenseTotalForceZ=off  SenseTotalTorque=off  SenseTotalTorqueX=off  SenseTotalTorqueY=off  SenseTotalTorqueZ=off  CompositeWrenchDir=FollowerOnBase  CompositeWrenchFrame=BaseFrame  PxEquilibriumPosition=0  PxEquilibriumPositionUnits=m  PxSpringStiffness=0  PxSpringStiffnessUnits=N/m  PxDampingCoefficient=b  PxDampingCoefficientUnits=N/(m/s)  PxTorqueActuationMode=NoTorque  PxMotionActuationMode=ComputedMotion  PxSensePosition=off  PxSenseVelocity=off  PxSenseAcceleration=off  PxSenseTorqueForce=off  PxSenseLowerLimitTorqueForce=off  PxSenseUpperLimitTorqueForce=off  PxLowerLimitSpecify=on  PxLowerLimitBound=-L/2  PxLowerLimitBoundUnits=m  PxLowerLimitStiffness=1e5  PxLowerLimitStiffnessUnits=N/m  PxLowerLimitDamping=sqrt(2e5)  PxLowerLimitDampingUnits=N/(m/s)  PxLowerLimitTransitionRegionWidth=1e-3  PxLowerLimitTransitionRegionWidthUnits=m  PxUpperLimitSpecify=on  PxUpperLimitBound=L/2  PxUpperLimitBoundUnits=m  PxUpperLimitStiffness=1e4  PxUpperLimitStiffnessUnits=N/m  PxUpperLimitDamping=sqrt(2e5)  PxUpperLimitDampingUnits=N/(m/s)  PxUpperLimitTransitionRegionWidth=1e-3  PxUpperLimitTransitionRegionWidthUnits=m  PxPositionTargetSpecify=on  PxPositionTargetPriority=High  PxPositionTargetValue=x0  PxPositionTargetValueUnits=m  PxVelocityTargetSpecify=off  PxVelocityTargetPriority=High  PxVelocityTargetValue=0  PxVelocityTargetValueUnits=m/s  PyEquilibriumPosition=0  PyEquilibriumPositionUnits=m  PySpringStiffness=0  PySpringStiffnessUnits=N/m  PyDampingCoefficient=b  PyDampingCoefficientUnits=N/(m/s)  PyTorqueActuationMode=NoTorque  PyMotionActuationMode=ComputedMotion  PySensePosition=off  PySenseVelocity=off  PySenseAcceleration=off  PySenseTorqueForce=off  PySenseLowerLimitTorqueForce=off  PySenseUpperLimitTorqueForce=off  PyLowerLimitSpecify=on  PyLowerLimitBound=-W/2  PyLowerLimitBoundUnits=m  PyLowerLimitStiffness=1e5  PyLowerLimitStiffnessUnits=N/m  PyLowerLimitDamping=sqrt(2e5)  PyLowerLimitDampingUnits=N/(m/s)  PyLowerLimitTransitionRegionWidth=1e-3  PyLowerLimitTransitionRegionWidthUnits=m  PyUpperLimitSpecify=on  PyUpperLimitBound=W/2  PyUpperLimitBoundUnits=m  PyUpperLimitStiffness=1e5  PyUpperLimitStiffnessUnits=N/m  PyUpperLimitDamping=sqrt(2e5)  PyUpperLimitDampingUnits=N/(m/s)  PyUpperLimitTransitionRegionWidth=1e-3  PyUpperLimitTransitionRegionWidthUnits=m  PyPositionTargetSpecify=on  PyPositionTargetPriority=High  PyPositionTargetValue=y0  PyPositionTargetValueUnits=m  PyVelocityTargetSpecify=off  PyVelocityTargetPriority=High  PyVelocityTargetValue=0  PyVelocityTargetValueUnits=m/s
  Spherical Solid : sm_lib/Body Elements/Spherical Solid  GraphicAmbientColor=[0.15 0.15 0.15 1.0]  BasedOnType=Density  CenterOfMass=[0 0 0]  CenterOfMassUnits=m  GraphicDiffuseColor=color  Density=1000  DensityUnits=kg/m^3  DoExposeReferenceFrame=on  GraphicEmissiveColor=[0.0 0.0 0.0 1.0]  ExportEntireGeometry=on  SerializedExposedGeometries=<ExposedGeometries><ExposedGeometry><RawGeometryId>entire</RawGeometryId><ExposedGeometryId>G</ExposedGeometryId></ExposedGeometry></ExposedGeometries>  SerializedFrames=<Frames/>  MarkerShape=Sphere  MarkerSize=10  GraphicType=FromGeometry  InertiaType=CalculateFromGeometry  Mass=1  MassUnits=kg  MomentsOfInertia=[1 1 1]  MomentsOfInertiaUnits=kg*m^2  GraphicOpacity=1.0  ProductsOfInertia=[0 0 0]  ProductsOfInertiaUnits=kg*m^2  GraphicShininess=75  GraphicSpecularColor=[0.5 0.5 0.5 1.0]  SphereRadius=R  SphereRadiusUnits=mm  GraphicVisPropType=SimpleVisualProperties
  WF : PMIOPort  Side=Left
  G : PMIOPort  Port=2  Side=Right
  R : PMIOPort  Port=3  Side=Left
  connections:
  Rectangular Joint/LConn1 -- WF/RConn1
  Spherical Solid/LConn1 -- G/RConn1
  Spherical Solid/RConn1 -- R/RConn1 -- Rectangular Joint/RConn1 -- External Force and Torque/RConn1
  PS Constant/RConn1 -- External Force and Torque/LConn1

== system ship_template/System/object scenario/3objs/objects/object location ==
  AND : Logic  Inputs=3  IconShape=distinctive  AllPortsSameDT=off  OutDataTypeStr=boolean
  Simscape Bus1 : SimscapeBus  HierarchyStrings=blue;green;red
  Stop Simulation : Stop
  World Frame : sm_lib/Frames and Transforms/World Frame
  checkCollected : Subsystem
  checkCollected1 : Subsystem
  checkCollected2 : Subsystem
  target vis : sm_lib/Body Elements/Revolved Solid  GraphicAmbientColor=[0.15 0.15 0.15 1.0]  BasedOnType=Density  CenterOfMass=[0 0 0]  CenterOfMassUnits=m  GraphicDiffuseColor=[0.8 0.0 0.2]  ExportConvexHullGeometry=off  Density=1000  DensityUnits=kg/m^3  DoExposeReferenceFrame=off  GraphicEmissiveColor=[0.0 0.0 0.0 1.0]  ExportEntireGeometry=off  SerializedFrames=<Frames><Frame><Id>Frame1</Id><Value><Name>F1</Name><Origin><Source>GeometricFeature</Source><FeatureName>side curve 1</FeatureName></Origin><PrimaryAxis><DefinedDirection>+Z</DefinedDirection><Source>ReferenceFrame</Source><SourceDirection>+Z</SourceDirection><FeatureName></FeatureName></PrimaryAxis><SecondaryAxis><DefinedDirection>+X</DefinedDirection><Source>ReferenceFrame</Source><SourceDirection>+X</SourceDirection><FeatureName></FeatureName></SecondaryAxis></Value></Frame></Frames>  MarkerShape=Sphere  MarkerSize=10  GraphicType=FromGeometry  InertiaType=CalculateFromGeometry  Mass=1  MassUnits=kg  MomentsOfInertia=[1 1 1]  MomentsOfInertiaUnits=kg*m^2  GraphicOpacity=1.0  ProductsOfInertia=[0 0 0]  ProductsOfInertiaUnits=kg*m^2  RevolutionCrossSection=homeRadius/2*[1.8 0.1; 1.8 -0.1; 2 -0.1; 2 0.1]  RevolutionCrossSectionUnits=m  RevolutionAngle=180  RevolutionAngleUnits=deg  RevolutionExtent=Full  GraphicShininess=75  GraphicSpecularColor=[0.5 0.5 0.5 1.0]  GraphicVisPropType=SimpleVisualProperties
  transform sensor : Subsystem
      settings: PortSchema="{\"entries\":[{\"content\":{\"sides\":[{\"content\":{\"connectorIds\":[\"LConn1\"]},\"type\":\"ConnectorPlacement.EquallySpacedRectSide\",\"uuid\":\"6f783dc6-d1fd-415b-a473-90d3874e8673\"},{\"content\":{\"connectorIds\":[\"RConn1\",\"Out1\"],\"side\":\"RIGHT\"},\"type\":\"ConnectorPlacement.EquallySpacedRectSide\",\"uuid\":\"5b02b9a2-9639-4136-ba9d-ee1490a18f64\"},{\"content\":{\"connectorIds\":[],\"side\":\"TOP\"},\"type\":\"ConnectorPlacement.EquallySpacedRectSide\",\"uuid\":\"b92e7d08-839c-4f34-a8a5-a6fd6b3e6ee4\"}]},\"type\":\"ConnectorPlacement.EquallySpacedConnector\",\"uuid\":\"bef9c973-2448-472f-911c-2cbdb1c4bcbd\"}],\"packageUris\":[\"http://schema.mathworks.com/mf0/Connector/R2020b\"],\"version\":\"1.0\"}"
  transform sensor1 : Subsystem
      settings: PortSchema="{\"entries\":[{\"content\":{\"sides\":[{\"content\":{\"connectorIds\":[\"LConn1\"]},\"type\":\"ConnectorPlacement.EquallySpacedRectSide\",\"uuid\":\"6f783dc6-d1fd-415b-a473-90d3874e8673\"},{\"content\":{\"connectorIds\":[\"RConn1\",\"Out1\"],\"side\":\"RIGHT\"},\"type\":\"ConnectorPlacement.EquallySpacedRectSide\",\"uuid\":\"5b02b9a2-9639-4136-ba9d-ee1490a18f64\"},{\"content\":{\"connectorIds\":[],\"side\":\"TOP\"},\"type\":\"ConnectorPlacement.EquallySpacedRectSide\",\"uuid\":\"b92e7d08-839c-4f34-a8a5-a6fd6b3e6ee4\"}]},\"type\":\"ConnectorPlacement.EquallySpacedConnector\",\"uuid\":\"bef9c973-2448-472f-911c-2cbdb1c4bcbd\"}],\"packageUris\":[\"http://schema.mathworks.com/mf0/Connector/R2020b\"],\"version\":\"1.0\"}"
  transform sensor2 : Subsystem
      settings: PortSchema="{\"entries\":[{\"content\":{\"sides\":[{\"content\":{\"connectorIds\":[\"LConn1\"]},\"type\":\"ConnectorPlacement.EquallySpacedRectSide\",\"uuid\":\"6f783dc6-d1fd-415b-a473-90d3874e8673\"},{\"content\":{\"connectorIds\":[\"RConn1\",\"Out1\"],\"side\":\"RIGHT\"},\"type\":\"ConnectorPlacement.EquallySpacedRectSide\",\"uuid\":\"5b02b9a2-9639-4136-ba9d-ee1490a18f64\"},{\"content\":{\"connectorIds\":[],\"side\":\"TOP\"},\"type\":\"ConnectorPlacement.EquallySpacedRectSide\",\"uuid\":\"b92e7d08-839c-4f34-a8a5-a6fd6b3e6ee4\"}]},\"type\":\"ConnectorPlacement.EquallySpacedConnector\",\"uuid\":\"bef9c973-2448-472f-911c-2cbdb1c4bcbd\"}],\"packageUris\":[\"http://schema.mathworks.com/mf0/Connector/R2020b\"],\"version\":\"1.0\"}"
  R : PMIOPort  Side=Right
  wires:
  AND/1 -> Stop Simulation/1  "allCollected"
  checkCollected/1(collectFlag) -> AND/1
  transform sensor/1(xy) -> checkCollected/1(xy)
  transform sensor1/1(xy) -> checkCollected1/1(xy)
  transform sensor2/1(xy) -> checkCollected2/1(xy)
  checkCollected1/1(collectFlag) -> AND/2
  checkCollected2/1(collectFlag) -> AND/3
  connections:
  Simscape Bus1/RConn1 -- R/RConn1
  World Frame/RConn1 -- transform sensor/LConn1 -- target vis/LConn1 -- transform sensor1/LConn1 -- transform sensor2/LConn1
  transform sensor/RConn1 -- Simscape Bus1/LConn1
  transform sensor1/RConn1 -- Simscape Bus1/LConn2
  transform sensor2/RConn1 -- Simscape Bus1/LConn3
